simulink model "MicrogridControl"  (R2025b)
settings: Solver=VariableStepAuto  StartTime=0.0  StopTime=8  FixedStep=Ts  RelTol=1e-3
PreLoadFcn:
  | NormalOperation;
  | MicrogridControlParam;
undefined symbols (not defined in the file): base, bessModeInitial, bessSystem, bessVoltage, breakerStatus, DiscIntNeverNeededParam, ee_sli_rtmsupport, event, gcbh, generator, gflInverter, gfmInverter, Inertia, lineInductance, lineResistance, machine, plannedIsland, pmsm, powerLimit, powerQuality, PV, PVInverter, ref, resync, solar, solarInsolationChange, systemFrequency, Ts, windController, windSystem, windTurbine
libraries: nesl_utility x234, ee_lib x174, fl_lib x143, eeGeneralControl x137, simulink x78, eeTransforms x47, slpidlib x23, nesl_utility_internal x12, eePwmGenerator x9, eeSinusoidalMeasurementV2 x9, custom_lib x7, batteryecm_lib x6
(part 19 of 25)

== system MicrogridControl/Wind Farm/Wind Plant Integrated/Detailed/Wind Turbine and Converters/Wind Controller/Machine Converter Control/Power Controller ==
  windSpeed : Inport
  Derating Control : Subsystem
  Greater than : simulink/Logic and Bit Operations/Compare To Constant  relop=>  const=12  OutDataTypeStr=boolean
  Less than or equal to : simulink/Logic and Bit Operations/Compare To Constant  relop=<=  const=12  OutDataTypeStr=boolean
  Limiter Function Power Demand : Subsystem
  MPPT Control : Subsystem
  activePowerDemand : Outport
  wires:
  Limiter Function Power Demand/1(activePowerDemand) -> activePowerDemand/1
  Derating Control/1(activePowerDemand) -> Limiter Function Power Demand/2(activePowerDemandDerating)
  MPPT Control/1(activePowerDemand) -> Limiter Function Power Demand/1(activePowerDemandMPPT)
  Greater than/1 -> Derating Control/Enable
  Less than or equal to/1 -> MPPT Control/Enable
  windSpeed/1 -> MPPT Control/1(windSpeed), Less than or equal to/1, Greater than/1

== system MicrogridControl/Wind Farm/Wind Plant Integrated/Detailed/Wind Turbine and Converters/Wind Controller/Machine Converter Control/Subsystem ==
  note: LVRT Crowbar Control
  Vdc : Inport
  LVRT : Inport  Port=2
  Abs : Abs  SaturateOnIntegerOverflow=off
  Constant1 : Constant  Value=Vdc
  Product : Product
  Relay : Relay  OnSwitchValue=0.01001*Vdc  OffSwitchValue=0.01*Vdc
  Sum : Sum  Inputs=|+-
  Unit Delay1 : UnitDelay  SampleTime=-1  HasFrameUpgradeWarning=on
  Out1 : Outport
  wires:
  Relay/1 -> Out1/1
  Product/1 -> Abs/1
  LVRT/1 -> Product/2
  Unit Delay1/1 -> Sum/2
  Abs/1 -> Relay/1
  Sum/1 -> Product/1
  Vdc/1 -> Unit Delay1/1
  Constant1/1 -> Sum/1

== system MicrogridControl/Wind Farm/Wind Plant Integrated/Detailed/Wind Turbine and Converters/Wind Controller/Wind Grid-side Converter Controller/Current_controller ==
  iWindd : Inport
  iq : Inport  Port=2
  id-ref : Inport  Port=3
  iqref : Inport  Port=4
  Vd : Inport  Port=5
  Vq : Inport  Port=6
  Constant4 : Constant  Value=0
  Gain1 : Gain  Gain=2*1*pi*frequency*inductance/baseImpedance
  Gain2 : Gain  Gain=2*1*pi*frequency*inductance/baseImpedance
  Mux1 : Mux  Inputs=3
  PI : Subsystem
  PI1 : Subsystem
  Sum1 : Sum  Inputs=|+-
  Sum3 : Sum  Inputs=|++-
  Sum4 : Sum  Inputs=|+++
  Sum5 : Sum  Inputs=|+-
  Refrence_mdq0 : Outport
  wires:
  Mux1/1 -> Refrence_mdq0/1  "m_dqo"
  Sum4/1 -> [Eq], Mux1/2
  PI1/1(Out2) -> Sum4/1
  iqref/1 -> Sum5/1
  Sum5/1 -> PI1/1(Input)
  Constant4/1 -> Mux1/3
  Vd/1 -> Sum3/1
  Sum1/1 -> PI/1(Input)
  iq/1 -> Sum5/2, Gain2/1
  Vq/1 -> Sum4/2
  Gain1/1 -> Sum4/3
  id-ref/1 -> Sum1/1
  iWindd/1 -> Sum1/2, Gain1/1
  Gain2/1 -> Sum3/3
  Sum3/1 -> [Ed], Mux1/1
  PI/1(Out2) -> Sum3/2

== system MicrogridControl/Wind Farm/Wind Plant Integrated/Detailed/Wind Turbine and Converters/Wind Controller/Wind Grid-side Converter Controller/DC Bus Chopper control  ==
  note: LVRT Detection
  In1 : Inport
  Constant1 : Constant
  Constant2 : Constant  Value=0
  Switch : Switch  Criteria=u2 > Threshold  Threshold=0.9  SaturateOnIntegerOverflow=off  InputSameDT=off
  Unit Delay : UnitDelay  SampleTime=-1  HasFrameUpgradeWarning=on
  Out1 : Outport
  wires:
  Unit Delay/1 -> Switch/2
  In1/1 -> Unit Delay/1
  Constant2/1 -> Switch/1
  Constant1/1 -> Switch/3
  Switch/1 -> Out1/1

== system MicrogridControl/Wind Farm/Wind Plant Integrated/Detailed/Wind Turbine and Converters/Wind Controller/Wind Grid-side Converter Controller/DC voltage controller & current reference ==
  note: id_ref_generator
  note: iq_ref_generator
  note: Limiter
  Q_ref : Inport
  Vmag : Inport  Port=2
  Wind_Mpp_vdc : Inport  Port=3
  Wind_vdc : Inport  Port=4
  lvrt.iq : Inport  Port=5
  Constant : Constant
  Constant1 : Constant  Value=iMaxPU
  Current limits : Subsystem
  Scope : Scope  NumInputPorts=2
      settings: ActiveDisplayYMinimum=-1  ActiveDisplayYMaximum=1  DataLoggingVariableName=ScopeData32
  Scope1 : Scope
      settings: ActiveDisplayYMinimum=-1  ActiveDisplayYMaximum=1  DataLoggingVariableName=ScopeData37
  Scope2 : Scope  NumInputPorts=2
      settings: ActiveDisplayYMinimum=-1  ActiveDisplayYMaximum=1  DataLoggingVariableName=ScopeData38
  Subsystem : Subsystem
  Subsystem1 : Subsystem
  Switch : Switch  Criteria=u2 > Threshold  SaturateOnIntegerOverflow=off  InputSameDT=off
  Unit Delay1 : UnitDelay  SampleTime=Ts  HasFrameUpgradeWarning=on
  Unit Delay3 : UnitDelay  SampleTime=Ts  HasFrameUpgradeWarning=on
  id_ref : Outport
  iq_ref : Outport  Port=2
  wires:
  Constant/1 -> Switch/3
  Switch/1 -> Scope1/1, Subsystem/1(V_mag)
  Vmag/1 -> Switch/2, Switch/1
  lvrt.iq/1 -> Subsystem/3(lvrt.iq)
  Current limits/1(iubq) -> Scope2/1, Subsystem/2(iq_ub)
  Wind_vdc/1 -> Scope/2, Subsystem1/2(Wind_vdc)
  Q_ref/1 -> Subsystem/4(Q_ref)
  Unit Delay3/1 -> Current limits/3(idref)
  Subsystem1/1(Out1) -> Unit Delay3/1, id_ref/1
  Unit Delay1/1 -> Current limits/2(iqref)
  Constant1/1 -> Current limits/1(Imax)
  Subsystem/1(Out1) -> iq_ref/1, Unit Delay1/1
  Current limits/2(iubd) -> Scope2/2, Subsystem1/3(id_ub)
  Wind_Mpp_vdc/1 -> Scope/1, Subsystem1/1(Wind_Mpp_vdc)

== system MicrogridControl/Wind Farm/Wind Plant Integrated/Detailed/Wind Turbine and Converters/Wind Plant/Back-to-Back Converters/Average ==
  Chopper : Inport
  SM_ref : Inport  Port=2
  Grid_ref : Inport  Port=3
  Capacitor : fl_lib/Electrical/Electrical Elements/Capacitor  c=capDC F  r=1e-1 Ohm  g=0 1/Ohm  i_specify=off  i_priority=None  i=0 A  i_nominal_specify=off  i_nominal_value=1  i_nominal_unit=A  v_specify=off  v_priority=None  v=0 V  v_nominal_specify=off  v_nominal_value=1  v_nominal_unit=V  vc_specify=on  vc_priority=None  vc=Vdc V  vc_nominal_specify=off  vc_nominal_value=1  vc_nominal_unit=V
  Electrical Reference : fl_lib/Electrical/Electrical Elements/Electrical Reference
  Electrical Reference1 : fl_lib/Electrical/Electrical Elements/Electrical Reference
  Electrical Reference2 : fl_lib/Electrical/Electrical Elements/Electrical Reference
  Grid Side Converter : ee_lib/Semiconductors & Converters/Converters/Average-Value Voltage Source Converter (Three-Phase)  port_option=ee.enum.threePhasePort.composite  frequency_option=ee.enum.converters.frequency.variable  input_option=ee.enum.converters.inputOption.ModWave  FRated=60 Hz  losses_parameterization=ee.enum.converters.losses.fixed  Pfixed=1 W  ks=0.01  kc1=1.7 V  kc2=0.01 Ohm  Ploss_vect=[100, 800, 1870, 3250, 4900] W  Irms_vect=[10, 100, 200, 300, 400] A  Vdc_nom=300 V  thermal_mass=30000 J/K  temperature_specify=off  temperature_priority=High  temperature=298.15 K  temperature_nominal_specify=off  temperature_nominal_value=1  temperature_nominal_unit=K
      settings: InternalSimscapePortConfiguration="{\"Bottom\":[],\"Left\":[{\"id\":\"ModWave\",\"label\":\"ModWave\",\"type\":\"input\"},{\"id\":\"N\",\"label\":\"~\",\"type\":\"foundation.electrical.three_phase\"}],\"Right\":[{\"id\":\"p\",\"label\":\"+\",\"type\":\"foundation.electrical.electrical\"},{\"id\":\"n\",\"label\":\"-\",\"type\":\"foundation.electrical.electrical\"}],\"Top\":[]}"
  Ideal Semiconductor Switch : ee_lib/Semiconductors & Converters/Ideal Semiconductor Switch  port_option=ee.enum.controlport.ps  Ron=0.001 Ohm  Goff=1e-6 1/Ohm  Vth=0.5 V  diode_param=ee.enum.converters.protectiondiode.none  diode_Vf=0.8 V  diode_Ron=0.001 Ohm  diode_Goff=1e-5 1/Ohm  diode_C=50e-9 F  diode_iRM=-235 A  diode_iF=300 A  diode_idot=-50 A/us  diode_trr_param=ee.enum.converters.diodetrr.trr_factor  diode_trr_factor=3  diode_trr=15 us  diode_Qrr=1500 s*uA
  Machine Side Converter : ee_lib/Semiconductors & Converters/Converters/Average-Value Voltage Source Converter (Three-Phase)  port_option=ee.enum.threePhasePort.composite  frequency_option=ee.enum.converters.frequency.variable  input_option=ee.enum.converters.inputOption.ModWave  FRated=60 Hz  losses_parameterization=ee.enum.converters.losses.fixed  Pfixed=1 W  ks=0.01  kc1=1.7 V  kc2=0.01 Ohm  Ploss_vect=[100, 800, 1870, 3250, 4900] W  Irms_vect=[10, 100, 200, 300, 400] A  Vdc_nom=300 V  thermal_mass=30000 J/K  temperature_specify=off  temperature_priority=High  temperature=298.15 K  temperature_nominal_specify=off  temperature_nominal_value=1  temperature_nominal_unit=K
      settings: InternalSimscapePortConfiguration="{\"Bottom\":[],\"Left\":[{\"id\":\"ModWave\",\"label\":\"ModWave\",\"type\":\"input\"},{\"id\":\"N\",\"label\":\"~\",\"type\":\"foundation.electrical.three_phase\"}],\"Right\":[{\"id\":\"p\",\"label\":\"+\",\"type\":\"foundation.electrical.electrical\"},{\"id\":\"n\",\"label\":\"-\",\"type\":\"foundation.electrical.electrical\"}],\"Top\":[]}"
  PS-Simulink Converter1 : nesl_utility/PS-Simulink Converter  PhysicalDomain=network_engine_domain  SubClassName=ps_output  LeftPortType=input  RightPortType=output  PseudoPeriodic=off  Frequencies=[]  VectorFormat=1-D array  Unit=V  AffineConversion=off
  Resistor : fl_lib/Electrical/Electrical Elements/Resistor  R=16 Ohm  i_specify=off  i_priority=None  i=0 A  i_nominal_specify=off  i_nominal_value=1  i_nominal_unit=A  v_specify=off  v_priority=None  v=0 V  v_nominal_specify=off  v_nominal_value=1  v_nominal_unit=V
  Scope : Scope
      settings: ActiveDisplayYMinimum=-0.125  ActiveDisplayYMaximum=1.125  DataLoggingVariableName=ScopeData11
  Simulink-PS Converter : nesl_utility/Simulink-PS Converter  PhysicalDomain=network_engine_domain  SubClassName=ps_input  LeftPortType=input  RightPortType=output  PseudoPeriodic=off  Frequencies=[]  NoiseDistribution=none  NoiseParameters=[]  Unit=1  AffineConversion=off  FilteringAndDerivatives=provide  SimscapeFilterOrder=1  InputFilterTimeConstant=0.001  UdotUserProvided=0
  Simulink-PS Converter2 : nesl_utility/Simulink-PS Converter  PhysicalDomain=network_engine_domain  SubClassName=ps_input  LeftPortType=input  RightPortType=output  PseudoPeriodic=off  Frequencies=[]  NoiseDistribution=none  NoiseParameters=[]  Unit=1  AffineConversion=off  FilteringAndDerivatives=provide  SimscapeFilterOrder=1  InputFilterTimeConstant=0.001  UdotUserProvided=0
  Simulink-PS Converter4 : nesl_utility/Simulink-PS Converter  PhysicalDomain=network_engine_domain  SubClassName=ps_input  LeftPortType=input  RightPortType=output  PseudoPeriodic=off  Frequencies=[]  NoiseDistribution=none  NoiseParameters=[]  Unit=1  AffineConversion=off  FilteringAndDerivatives=provide  SimscapeFilterOrder=1  InputFilterTimeConstant=0.001  UdotUserProvided=0
  Voltage Sensor : fl_lib/Electrical/Electrical Sensors/Voltage Sensor
  In : PMIOPort  Side=Left
  ~ : PMIOPort  Port=2  Side=Right
  Vdc : Outport
  wires:
  SM_ref/1 -> Simulink-PS Converter/1
  PS-Simulink Converter1/1 -> Vdc/1  "Vdc"
  Chopper/1 -> Simulink-PS Converter2/1, Scope/1
  Grid_ref/1 -> Simulink-PS Converter4/1
  connections:
  Simulink-PS Converter/RConn1 -- Machine Side Converter/LConn1
  Machine Side Converter/LConn2 -- In/RConn1
  Simulink-PS Converter2/RConn1 -- Ideal Semiconductor Switch/LConn1
  Electrical Reference1/LConn1 -- Resistor/RConn1
  Grid Side Converter/LConn1 -- Simulink-PS Converter4/RConn1
  Resistor/LConn1 -- Ideal Semiconductor Switch/RConn2
  ~/RConn1 -- Grid Side Converter/LConn2
  PS-Simulink Converter1/LConn1 -- Voltage Sensor/RConn1
  Electrical Reference2/LConn1 -- Grid Side Converter/RConn2
  Voltage Sensor/LConn1 -- Machine Side Converter/RConn1 -- Ideal Semiconductor Switch/RConn1 -- Grid Side Converter/RConn1 -- Capacitor/LConn1
  Capacitor/RConn1 -- Voltage Sensor/RConn2 -- Machine Side Converter/RConn2 -- Electrical Reference/LConn1

== system MicrogridControl/Wind Farm/Wind Plant Integrated/Detailed/Wind Turbine and Converters/Wind Plant/Back-to-Back Converters/Switching ==
  Chopper : Inport
  SM_ref : Inport  Port=2
  Grid_ref : Inport  Port=3
  Capacitor : fl_lib/Electrical/Electrical Elements/Capacitor  c=capacitance F  r=1e-1 Ohm  g=0 1/Ohm  i_specify=off  i_priority=None  i=0 A  i_nominal_specify=off  i_nominal_value=1  i_nominal_unit=A  v_specify=off  v_priority=None  v=0 V  v_nominal_specify=off  v_nominal_value=1  v_nominal_unit=V  vc_specify=on  vc_priority=High  vc=baseVoltageDC V  vc_nominal_specify=off  vc_nominal_value=1  vc_nominal_unit=V
  Electrical Reference : fl_lib/Electrical/Electrical Elements/Electrical Reference
  Electrical Reference1 : fl_lib/Electrical/Electrical Elements/Electrical Reference
  Electrical Reference2 : fl_lib/Electrical/Electrical Elements/Electrical Reference
  Grid Side Converter : Subsystem
      settings: PortSchema="{\"entries\":[{\"content\":{\"sides\":[{\"content\":{\"connectorIds\":[\"LConn1\",\"LConn2\"]},\"type\":\"ConnectorPlacement.EquallySpacedRectSide\",\"uuid\":\"e32be008-cebd-46aa-ba62-c5c92b9b23e3\"},{\"content\":{\"connectorIds\":[\"In1\",\"RConn1\"],\"side\":\"RIGHT\"},\"type\":\"ConnectorPlacement.EquallySpacedRectSide\",\"uuid\":\"c483e451-04b5-4212-bdd1-c589ba5bea78\"},{\"content\":{\"side\":\"TOP\"},\"type\":\"ConnectorPlacement.EquallySpacedRectSide\",\"uuid\":\"824c135c-7e5f-4da0-a7de-e626b4bfa50d\"}]},\"type\":\"ConnectorPlacement.EquallySpacedConnector\",\"uuid\":\"5f81c72d-92ab-4525-91a6-193f769a7c86\"}],\"packageUris\":[\"http://schema.mathworks.com/mf0/Connector/R2020b\"],\"version\":\"1.0\"}"
  Ideal Semiconductor Switch : ee_lib/Semiconductors & Converters/Ideal Semiconductor Switch  port_option=ee.enum.controlport.ps  Ron=0.001 Ohm  Goff=1e-6 1/Ohm  Vth=0.5 V  diode_param=ee.enum.converters.protectiondiode.none  diode_Vf=0.8 V  diode_Ron=0.001 Ohm  diode_Goff=1e-5 1/Ohm  diode_C=50e-9 F  diode_iRM=-235 A  diode_iF=300 A  diode_idot=-50 A/us  diode_trr_param=ee.enum.converters.diodetrr.trr_factor  diode_trr_factor=3  diode_trr=15 us  diode_Qrr=1500 s*uA
  Machine Side Converter : Subsystem
      settings: PortSchema="{\"entries\":[{\"content\":{\"sides\":[{\"content\":{\"connectorIds\":[\"LConn1\",\"LConn2\"]},\"type\":\"ConnectorPlacement.EquallySpacedRectSide\",\"uuid\":\"e32be008-cebd-46aa-ba62-c5c92b9b23e3\"},{\"content\":{\"connectorIds\":[\"In1\",\"RConn1\"],\"side\":\"RIGHT\"},\"type\":\"ConnectorPlacement.EquallySpacedRectSide\",\"uuid\":\"c483e451-04b5-4212-bdd1-c589ba5bea78\"},{\"content\":{\"side\":\"TOP\"},\"type\":\"ConnectorPlacement.EquallySpacedRectSide\",\"uuid\":\"824c135c-7e5f-4da0-a7de-e626b4bfa50d\"}]},\"type\":\"ConnectorPlacement.EquallySpacedConnector\",\"uuid\":\"5f81c72d-92ab-4525-91a6-193f769a7c86\"}],\"packageUris\":[\"http://schema.mathworks.com/mf0/Connector/R2020b\"],\"version\":\"1.0\"}"
  PS-Simulink Converter1 : nesl_utility/PS-Simulink Converter  PhysicalDomain=network_engine_domain  SubClassName=ps_output  LeftPortType=input  RightPortType=output  PseudoPeriodic=off  Frequencies=[]  VectorFormat=1-D array  Unit=V  AffineConversion=off
  Resistor : fl_lib/Electrical/Electrical Elements/Resistor  R=16 Ohm  i_specify=off  i_priority=None  i=0 A  i_nominal_specify=off  i_nominal_value=1  i_nominal_unit=A  v_specify=off  v_priority=None  v=0 V  v_nominal_specify=off  v_nominal_value=1  v_nominal_unit=V
  Scope : Scope
      settings: ActiveDisplayYMinimum=-0.125  ActiveDisplayYMaximum=1.125  DataLoggingVariableName=ScopeData11
  Simulink-PS Converter2 : nesl_utility/Simulink-PS Converter  PhysicalDomain=network_engine_domain  SubClassName=ps_input  LeftPortType=input  RightPortType=output  PseudoPeriodic=off  Frequencies=[]  NoiseDistribution=none  NoiseParameters=[]  Unit=1  AffineConversion=off  FilteringAndDerivatives=provide  SimscapeFilterOrder=1  InputFilterTimeConstant=0.001  UdotUserProvided=0
  Voltage Sensor : fl_lib/Electrical/Electrical Sensors/Voltage Sensor
  In : PMIOPort  Side=Left
  ~ : PMIOPort  Port=2  Side=Right
  Vdc : Outport
  wires:
  PS-Simulink Converter1/1 -> Vdc/1  "Vdc"
  Chopper/1 -> Simulink-PS Converter2/1, Scope/1
  Grid_ref/1 -> Grid Side Converter/1(mabc)
  SM_ref/1 -> Machine Side Converter/1(mabc)
  connections:
  Machine Side Converter/RConn1 -- In/RConn1
  Simulink-PS Converter2/RConn1 -- Ideal Semiconductor Switch/LConn1
  Electrical Reference1/LConn1 -- Resistor/RConn1
  Resistor/LConn1 -- Ideal Semiconductor Switch/RConn2
  ~/RConn1 -- Grid Side Converter/RConn1
  PS-Simulink Converter1/LConn1 -- Voltage Sensor/RConn1
  Grid Side Converter/LConn2 -- Electrical Reference2/LConn1
  Voltage Sensor/LConn1 -- Machine Side Converter/LConn1 -- Capacitor/LConn1 -- Grid Side Converter/LConn1 -- Ideal Semiconductor Switch/RConn1
  Electrical Reference/LConn1 -- Voltage Sensor/RConn2 -- Machine Side Converter/LConn2 -- Capacitor/RConn1

== system MicrogridControl/Wind Farm/Wind Plant Integrated1/Detailed/Wind Turbine and Converters/Wind Controller/Machine Converter Control/Measurements ==
  iabc_sens : Inport
  w_sens : Inport  Port=2
  th_sens : Inport  Port=3
  Vdc_sens : Inport  Port=4
  2*pi : Constant  Value=2*pi  SampleTime=-1
  Math Function : Math  Operator=mod  SignedPower=on
  pole pairs : Gain  Gain=p
  "pole pairs " : Gain  Gain=p
  we : Outport  VectorParamsAs1DForOutWhenUnconnected=off
  iabc : Outport  Port=2  VectorParamsAs1DForOutWhenUnconnected=off
  theta : Outport  Port=3  VectorParamsAs1DForOutWhenUnconnected=off
  Vdc : Outport  Port=4  VectorParamsAs1DForOutWhenUnconnected=off
  wires:
  Math Function/1 -> theta/1
  Vdc_sens/1 -> Vdc/1
  "pole pairs "/1 -> Math Function/1
  th_sens/1 -> "pole pairs "/1
  2*pi/1 -> Math Function/2
  pole pairs/1 -> we/1
  iabc_sens/1 -> iabc/1
  w_sens/1 -> pole pairs/1

== system MicrogridControl/Wind Farm/Wind Plant Integrated1/Detailed/Wind Turbine and Converters/Wind Controller/Machine Converter Control/Power Controller ==
  windSpeed : Inport
  Derating Control : Subsystem
  Greater than : simulink/Logic and Bit Operations/Compare To Constant  relop=>  const=12  OutDataTypeStr=boolean
  Less than or equal to : simulink/Logic and Bit Operations/Compare To Constant  relop=<=  const=12  OutDataTypeStr=boolean
  Limiter Function Power Demand : Subsystem
  MPPT Control : Subsystem
  activePowerDemand : Outport
  wires:
  Limiter Function Power Demand/1(activePowerDemand) -> activePowerDemand/1
  Derating Control/1(activePowerDemand) -> Limiter Function Power Demand/2(activePowerDemandDerating)
  MPPT Control/1(activePowerDemand) -> Limiter Function Power Demand/1(activePowerDemandMPPT)
  Greater than/1 -> Derating Control/Enable
  Less than or equal to/1 -> MPPT Control/Enable
  windSpeed/1 -> MPPT Control/1(windSpeed), Less than or equal to/1, Greater than/1

== system MicrogridControl/Wind Farm/Wind Plant Integrated1/Detailed/Wind Turbine and Converters/Wind Controller/Machine Converter Control/Subsystem ==
  note: LVRT Crowbar Control
  Vdc : Inport
  LVRT : Inport  Port=2
  Abs : Abs  SaturateOnIntegerOverflow=off
  Constant1 : Constant  Value=Vdc
  Product : Product
  Relay : Relay  OnSwitchValue=0.01001*Vdc  OffSwitchValue=0.01*Vdc
  Sum : Sum  Inputs=|+-
  Unit Delay1 : UnitDelay  SampleTime=-1  HasFrameUpgradeWarning=on
  Out1 : Outport
  wires:
  Relay/1 -> Out1/1
  Product/1 -> Abs/1
  LVRT/1 -> Product/2
  Unit Delay1/1 -> Sum/2
  Abs/1 -> Relay/1
  Sum/1 -> Product/1
  Vdc/1 -> Unit Delay1/1
  Constant1/1 -> Sum/1

== system MicrogridControl/Wind Farm/Wind Plant Integrated1/Detailed/Wind Turbine and Converters/Wind Controller/Wind Grid-side Converter Controller/Current_controller ==
  iWindd : Inport
  iq : Inport  Port=2
  id-ref : Inport  Port=3
  iqref : Inport  Port=4
  Vd : Inport  Port=5
  Vq : Inport  Port=6
  Constant4 : Constant  Value=0
  Gain1 : Gain  Gain=2*1*pi*frequency*inductance/baseImpedance
  Gain2 : Gain  Gain=2*1*pi*frequency*inductance/baseImpedance
  Mux1 : Mux  Inputs=3
  PI : Subsystem
  PI1 : Subsystem
  Sum1 : Sum  Inputs=|+-
  Sum3 : Sum  Inputs=|++-
  Sum4 : Sum  Inputs=|+++
  Sum5 : Sum  Inputs=|+-
  Refrence_mdq0 : Outport
  wires:
  Mux1/1 -> Refrence_mdq0/1  "m_dqo"
  Sum4/1 -> [Eq], Mux1/2
  PI1/1(Out2) -> Sum4/1
  iqref/1 -> Sum5/1
  Sum5/1 -> PI1/1(Input)
  Constant4/1 -> Mux1/3
  Vd/1 -> Sum3/1
  Sum1/1 -> PI/1(Input)
  iq/1 -> Sum5/2, Gain2/1
  Vq/1 -> Sum4/2
  Gain1/1 -> Sum4/3
  id-ref/1 -> Sum1/1
  iWindd/1 -> Sum1/2, Gain1/1
  Gain2/1 -> Sum3/3
  Sum3/1 -> [Ed], Mux1/1
  PI/1(Out2) -> Sum3/2

== system MicrogridControl/Wind Farm/Wind Plant Integrated1/Detailed/Wind Turbine and Converters/Wind Controller/Wind Grid-side Converter Controller/DC Bus Chopper control  ==
  note: LVRT Detection
  In1 : Inport
  Constant1 : Constant
  Constant2 : Constant  Value=0
  Switch : Switch  Criteria=u2 > Threshold  Threshold=0.9  SaturateOnIntegerOverflow=off  InputSameDT=off
  Unit Delay : UnitDelay  SampleTime=-1  HasFrameUpgradeWarning=on
  Out1 : Outport
  wires:
  Unit Delay/1 -> Switch/2
  In1/1 -> Unit Delay/1
  Constant2/1 -> Switch/1
  Constant1/1 -> Switch/3
  Switch/1 -> Out1/1

== system MicrogridControl/Wind Farm/Wind Plant Integrated1/Detailed/Wind Turbine and Converters/Wind Controller/Wind Grid-side Converter Controller/DC voltage controller & current reference ==
  note: id_ref_generator
  note: iq_ref_generator
  note: Limiter
  Q_ref : Inport
  Vmag : Inport  Port=2
  Wind_Mpp_vdc : Inport  Port=3
  Wind_vdc : Inport  Port=4
  lvrt.iq : Inport  Port=5
  Constant : Constant
  Constant1 : Constant  Value=iMaxPU
  Current limits : Subsystem
  Subsystem : Subsystem
  Subsystem1 : Subsystem
  Switch : Switch  Criteria=u2 > Threshold  SaturateOnIntegerOverflow=off  InputSameDT=off
  Unit Delay1 : UnitDelay  SampleTime=Ts  HasFrameUpgradeWarning=on
  Unit Delay3 : UnitDelay  SampleTime=Ts  HasFrameUpgradeWarning=on
  id_ref : Outport
  iq_ref : Outport  Port=2
  wires:
  Constant/1 -> Switch/3
  Switch/1 -> Subsystem/1(V_mag)
  Vmag/1 -> Switch/2, Switch/1
  lvrt.iq/1 -> Subsystem/3(lvrt.iq)
  Current limits/1(iubq) -> Subsystem/2(iq_ub)
  Wind_vdc/1 -> Subsystem1/2(Wind_vdc)
  Wind_Mpp_vdc/1 -> Subsystem1/1(Wind_Mpp_vdc)
  Q_ref/1 -> Subsystem/4(Q_ref)
  Unit Delay3/1 -> Current limits/3(idref)
  Subsystem1/1(Out1) -> Unit Delay3/1, id_ref/1
  Unit Delay1/1 -> Current limits/2(iqref)
  Constant1/1 -> Current limits/1(Imax)
  Subsystem/1(Out1) -> iq_ref/1, Unit Delay1/1
  Current limits/2(iubd) -> Subsystem1/3(id_ub)

== system MicrogridControl/Wind Farm/Wind Plant Integrated1/Detailed/Wind Turbine and Converters/Wind Plant/Back-to-Back Converters/Average ==
  Chopper : Inport
  SM_ref : Inport  Port=2
  Grid_ref : Inport  Port=3
  Capacitor : fl_lib/Electrical/Electrical Elements/Capacitor  c=capDC F  r=1e-1 Ohm  g=0 1/Ohm  i_specify=off  i_priority=None  i=0 A  i_nominal_specify=off  i_nominal_value=1  i_nominal_unit=A  v_specify=off  v_priority=None  v=0 V  v_nominal_specify=off  v_nominal_value=1  v_nominal_unit=V  vc_specify=on  vc_priority=None  vc=Vdc V  vc_nominal_specify=off  vc_nominal_value=1  vc_nominal_unit=V
  Electrical Reference : fl_lib/Electrical/Electrical Elements/Electrical Reference
  Electrical Reference1 : fl_lib/Electrical/Electrical Elements/Electrical Reference
  Electrical Reference2 : fl_lib/Electrical/Electrical Elements/Electrical Reference
  Grid Side Converter : ee_lib/Semiconductors & Converters/Converters/Average-Value Voltage Source Converter (Three-Phase)  port_option=ee.enum.threePhasePort.composite  frequency_option=ee.enum.converters.frequency.variable  input_option=ee.enum.converters.inputOption.ModWave  FRated=60 Hz  losses_parameterization=ee.enum.converters.losses.fixed  Pfixed=1 W  ks=0.01  kc1=1.7 V  kc2=0.01 Ohm  Ploss_vect=[100, 800, 1870, 3250, 4900] W  Irms_vect=[10, 100, 200, 300, 400] A  Vdc_nom=300 V  thermal_mass=30000 J/K  temperature_specify=off  temperature_priority=High  temperature=298.15 K  temperature_nominal_specify=off  temperature_nominal_value=1  temperature_nominal_unit=K
      settings: InternalSimscapePortConfiguration="{\"Bottom\":[],\"Left\":[{\"id\":\"ModWave\",\"label\":\"ModWave\",\"type\":\"input\"},{\"id\":\"N\",\"label\":\"~\",\"type\":\"foundation.electrical.three_phase\"}],\"Right\":[{\"id\":\"p\",\"label\":\"+\",\"type\":\"foundation.electrical.electrical\"},{\"id\":\"n\",\"label\":\"-\",\"type\":\"foundation.electrical.electrical\"}],\"Top\":[]}"
  Ideal Semiconductor Switch : ee_lib/Semiconductors & Converters/Ideal Semiconductor Switch  port_option=ee.enum.controlport.ps  Ron=0.001 Ohm  Goff=1e-6 1/Ohm  Vth=0.5 V  diode_param=ee.enum.converters.protectiondiode.none  diode_Vf=0.8 V  diode_Ron=0.001 Ohm  diode_Goff=1e-5 1/Ohm  diode_C=50e-9 F  diode_iRM=-235 A  diode_iF=300 A  diode_idot=-50 A/us  diode_trr_param=ee.enum.converters.diodetrr.trr_factor  diode_trr_factor=3  diode_trr=15 us  diode_Qrr=1500 s*uA
  Machine Side Converter : ee_lib/Semiconductors & Converters/Converters/Average-Value Voltage Source Converter (Three-Phase)  port_option=ee.enum.threePhasePort.composite  frequency_option=ee.enum.converters.frequency.variable  input_option=ee.enum.converters.inputOption.ModWave  FRated=60 Hz  losses_parameterization=ee.enum.converters.losses.fixed  Pfixed=1 W  ks=0.01  kc1=1.7 V  kc2=0.01 Ohm  Ploss_vect=[100, 800, 1870, 3250, 4900] W  Irms_vect=[10, 100, 200, 300, 400] A  Vdc_nom=300 V  thermal_mass=30000 J/K  temperature_specify=off  temperature_priority=High  temperature=298.15 K  temperature_nominal_specify=off  temperature_nominal_value=1  temperature_nominal_unit=K
      settings: InternalSimscapePortConfiguration="{\"Bottom\":[],\"Left\":[{\"id\":\"ModWave\",\"label\":\"ModWave\",\"type\":\"input\"},{\"id\":\"N\",\"label\":\"~\",\"type\":\"foundation.electrical.three_phase\"}],\"Right\":[{\"id\":\"p\",\"label\":\"+\",\"type\":\"foundation.electrical.electrical\"},{\"id\":\"n\",\"label\":\"-\",\"type\":\"foundation.electrical.electrical\"}],\"Top\":[]}"
  PS-Simulink Converter1 : nesl_utility/PS-Simulink Converter  PhysicalDomain=network_engine_domain  SubClassName=ps_output  LeftPortType=input  RightPortType=output  PseudoPeriodic=off  Frequencies=[]  VectorFormat=1-D array  Unit=V  AffineConversion=off
  Resistor : fl_lib/Electrical/Electrical Elements/Resistor  R=16 Ohm  i_specify=off  i_priority=None  i=0 A  i_nominal_specify=off  i_nominal_value=1  i_nominal_unit=A  v_specify=off  v_priority=None  v=0 V  v_nominal_specify=off  v_nominal_value=1  v_nominal_unit=V
  Scope : Scope
      settings: ActiveDisplayYMinimum=-0.125  ActiveDisplayYMaximum=1.125  DataLoggingVariableName=ScopeData11
  Simulink-PS Converter : nesl_utility/Simulink-PS Converter  PhysicalDomain=network_engine_domain  SubClassName=ps_input  LeftPortType=input  RightPortType=output  PseudoPeriodic=off  Frequencies=[]  NoiseDistribution=none  NoiseParameters=[]  Unit=1  AffineConversion=off  FilteringAndDerivatives=provide  SimscapeFilterOrder=1  InputFilterTimeConstant=0.001  UdotUserProvided=0
  Simulink-PS Converter2 : nesl_utility/Simulink-PS Converter  PhysicalDomain=network_engine_domain  SubClassName=ps_input  LeftPortType=input  RightPortType=output  PseudoPeriodic=off  Frequencies=[]  NoiseDistribution=none  NoiseParameters=[]  Unit=1  AffineConversion=off  FilteringAndDerivatives=provide  SimscapeFilterOrder=1  InputFilterTimeConstant=0.001  UdotUserProvided=0
  Simulink-PS Converter4 : nesl_utility/Simulink-PS Converter  PhysicalDomain=network_engine_domain  SubClassName=ps_input  LeftPortType=input  RightPortType=output  PseudoPeriodic=off  Frequencies=[]  NoiseDistribution=none  NoiseParameters=[]  Unit=1  AffineConversion=off  FilteringAndDerivatives=provide  SimscapeFilterOrder=1  InputFilterTimeConstant=0.001  UdotUserProvided=0
  Voltage Sensor : fl_lib/Electrical/Electrical Sensors/Voltage Sensor
  In : PMIOPort  Side=Left
  ~ : PMIOPort  Port=2  Side=Right
  Vdc : Outport
  wires:
  SM_ref/1 -> Simulink-PS Converter/1
  PS-Simulink Converter1/1 -> Vdc/1  "Vdc"
  Chopper/1 -> Simulink-PS Converter2/1, Scope/1
  Grid_ref/1 -> Simulink-PS Converter4/1
  connections:
  Simulink-PS Converter/RConn1 -- Machine Side Converter/LConn1
  Machine Side Converter/LConn2 -- In/RConn1
  Simulink-PS Converter2/RConn1 -- Ideal Semiconductor Switch/LConn1
  Electrical Reference1/LConn1 -- Resistor/RConn1
  Grid Side Converter/LConn1 -- Simulink-PS Converter4/RConn1
  Resistor/LConn1 -- Ideal Semiconductor Switch/RConn2
  ~/RConn1 -- Grid Side Converter/LConn2
  PS-Simulink Converter1/LConn1 -- Voltage Sensor/RConn1
  Electrical Reference2/LConn1 -- Grid Side Converter/RConn2
  Voltage Sensor/LConn1 -- Machine Side Converter/RConn1 -- Ideal Semiconductor Switch/RConn1 -- Grid Side Converter/RConn1 -- Capacitor/LConn1
  Capacitor/RConn1 -- Voltage Sensor/RConn2 -- Machine Side Converter/RConn2 -- Electrical Reference/LConn1

== system MicrogridControl/Wind Farm/Wind Plant Integrated1/Detailed/Wind Turbine and Converters/Wind Plant/Back-to-Back Converters/Switching ==
  Chopper : Inport
  SM_ref : Inport  Port=2
  Grid_ref : Inport  Port=3
  Capacitor : fl_lib/Electrical/Electrical Elements/Capacitor  c=capacitance F  r=1e-1 Ohm  g=0 1/Ohm  i_specify=off  i_priority=None  i=0 A  i_nominal_specify=off  i_nominal_value=1  i_nominal_unit=A  v_specify=off  v_priority=None  v=0 V  v_nominal_specify=off  v_nominal_value=1  v_nominal_unit=V  vc_specify=on  vc_priority=High  vc=baseVoltageDC V  vc_nominal_specify=off  vc_nominal_value=1  vc_nominal_unit=V
  Electrical Reference : fl_lib/Electrical/Electrical Elements/Electrical Reference
  Electrical Reference1 : fl_lib/Electrical/Electrical Elements/Electrical Reference
  Electrical Reference2 : fl_lib/Electrical/Electrical Elements/Electrical Reference
  Grid Side Converter : Subsystem
      settings: PortSchema="{\"entries\":[{\"content\":{\"sides\":[{\"content\":{\"connectorIds\":[\"LConn1\",\"LConn2\"]},\"type\":\"ConnectorPlacement.EquallySpacedRectSide\",\"uuid\":\"e32be008-cebd-46aa-ba62-c5c92b9b23e3\"},{\"content\":{\"connectorIds\":[\"In1\",\"RConn1\"],\"side\":\"RIGHT\"},\"type\":\"ConnectorPlacement.EquallySpacedRectSide\",\"uuid\":\"c483e451-04b5-4212-bdd1-c589ba5bea78\"},{\"content\":{\"side\":\"TOP\"},\"type\":\"ConnectorPlacement.EquallySpacedRectSide\",\"uuid\":\"824c135c-7e5f-4da0-a7de-e626b4bfa50d\"}]},\"type\":\"ConnectorPlacement.EquallySpacedConnector\",\"uuid\":\"5f81c72d-92ab-4525-91a6-193f769a7c86\"}],\"packageUris\":[\"http://schema.mathworks.com/mf0/Connector/R2020b\"],\"version\":\"1.0\"}"
  Ideal Semiconductor Switch : ee_lib/Semiconductors & Converters/Ideal Semiconductor Switch  port_option=ee.enum.controlport.ps  Ron=0.001 Ohm  Goff=1e-6 1/Ohm  Vth=0.5 V  diode_param=ee.enum.converters.protectiondiode.none  diode_Vf=0.8 V  diode_Ron=0.001 Ohm  diode_Goff=1e-5 1/Ohm  diode_C=50e-9 F  diode_iRM=-235 A  diode_iF=300 A  diode_idot=-50 A/us  diode_trr_param=ee.enum.converters.diodetrr.trr_factor  diode_trr_factor=3  diode_trr=15 us  diode_Qrr=1500 s*uA
  Machine Side Converter : Subsystem
      settings: PortSchema="{\"entries\":[{\"content\":{\"sides\":[{\"content\":{\"connectorIds\":[\"LConn1\",\"LConn2\"]},\"type\":\"ConnectorPlacement.EquallySpacedRectSide\",\"uuid\":\"e32be008-cebd-46aa-ba62-c5c92b9b23e3\"},{\"content\":{\"connectorIds\":[\"In1\",\"RConn1\"],\"side\":\"RIGHT\"},\"type\":\"ConnectorPlacement.EquallySpacedRectSide\",\"uuid\":\"c483e451-04b5-4212-bdd1-c589ba5bea78\"},{\"content\":{\"side\":\"TOP\"},\"type\":\"ConnectorPlacement.EquallySpacedRectSide\",\"uuid\":\"824c135c-7e5f-4da0-a7de-e626b4bfa50d\"}]},\"type\":\"ConnectorPlacement.EquallySpacedConnector\",\"uuid\":\"5f81c72d-92ab-4525-91a6-193f769a7c86\"}],\"packageUris\":[\"http://schema.mathworks.com/mf0/Connector/R2020b\"],\"version\":\"1.0\"}"
  PS-Simulink Converter1 : nesl_utility/PS-Simulink Converter  PhysicalDomain=network_engine_domain  SubClassName=ps_output  LeftPortType=input  RightPortType=output  PseudoPeriodic=off  Frequencies=[]  VectorFormat=1-D array  Unit=V  AffineConversion=off
  Resistor : fl_lib/Electrical/Electrical Elements/Resistor  R=16 Ohm  i_specify=off  i_priority=None  i=0 A  i_nominal_specify=off  i_nominal_value=1  i_nominal_unit=A  v_specify=off  v_priority=None  v=0 V  v_nominal_specify=off  v_nominal_value=1  v_nominal_unit=V
  Scope : Scope
      settings: ActiveDisplayYMinimum=-0.125  ActiveDisplayYMaximum=1.125  DataLoggingVariableName=ScopeData11
  Simulink-PS Converter2 : nesl_utility/Simulink-PS Converter  PhysicalDomain=network_engine_domain  SubClassName=ps_input  LeftPortType=input  RightPortType=output  PseudoPeriodic=off  Frequencies=[]  NoiseDistribution=none  NoiseParameters=[]  Unit=1  AffineConversion=off  FilteringAndDerivatives=provide  SimscapeFilterOrder=1  InputFilterTimeConstant=0.001  UdotUserProvided=0
  Voltage Sensor : fl_lib/Electrical/Electrical Sensors/Voltage Sensor
  In : PMIOPort  Side=Left
  ~ : PMIOPort  Port=2  Side=Right
  Vdc : Outport
  wires:
  PS-Simulink Converter1/1 -> Vdc/1  "Vdc"
  Chopper/1 -> Simulink-PS Converter2/1, Scope/1
  Grid_ref/1 -> Grid Side Converter/1(mabc)
  SM_ref/1 -> Machine Side Converter/1(mabc)
  connections:
  Machine Side Converter/RConn1 -- In/RConn1
  Simulink-PS Converter2/RConn1 -- Ideal Semiconductor Switch/LConn1
  Electrical Reference1/LConn1 -- Resistor/RConn1
  Resistor/LConn1 -- Ideal Semiconductor Switch/RConn2
  ~/RConn1 -- Grid Side Converter/RConn1
  PS-Simulink Converter1/LConn1 -- Voltage Sensor/RConn1
  Grid Side Converter/LConn2 -- Electrical Reference2/LConn1
  Voltage Sensor/LConn1 -- Machine Side Converter/LConn1 -- Capacitor/LConn1 -- Grid Side Converter/LConn1 -- Ideal Semiconductor Switch/RConn1
  Electrical Reference/LConn1 -- Voltage Sensor/RConn2 -- Machine Side Converter/LConn2 -- Capacitor/RConn1

== system MicrogridControl/BESS/BESS Integrated/Detailed/BESS Controller/Grid Forming/Current Limiting/CurrentLimitingMethod/currentLimitAndVirtual ==
  Igd : Inport
  Igq : Inport  Port=2
  Current Saturation : Subsystem
  CurrentLimitSelection : Stateflow chart  TreatAsAtomicUnit=on
  Math Function : Math  Operator=hypot
  Merge{,1..3} (4 alike) : Merge  Inputs=3
  No Fault Ride Through : Subsystem
  VI : Subsystem
  delVd : Outport
  delVq : Outport  Port=2
  Idmax : Outport  Port=3
  Iqmax : Outport  Port=4
  wires:
  [Imax] -> VI/3(Imax)
  [Imax] -> Current Saturation/3(Imaxsat)
  [noCtLt] -> No Fault Ride Through/Enable
  [satCtLt] -> Current Saturation/Enable
  [viCtLt] -> VI/Enable
  CurrentLimitSelection/4(satCurrentLimit) -> [satCtLt]
  CurrentLimitSelection/3(viCurrentLimit) -> [viCtLt]
  CurrentLimitSelection/2(noCurrentLimit) -> [noCtLt]
  CurrentLimitSelection/1(ismax) -> [Imax]
  Math Function/1 -> CurrentLimitSelection/1(Is)
  No Fault Ride Through/2(delVq) -> Merge1/3
  Merge3/1 -> Iqmax/1
  Current Saturation/2(delVq) -> Merge1/2
  No Fault Ride Through/4(iqmax) -> Merge3/3
  VI/3(idmax) -> Merge2/1
  VI/4(iqmax) -> Merge3/1
  Current Saturation/3(idmax) -> Merge2/2
  VI/2(delVq) -> Merge1/1
  Merge/1 -> delVd/1
  Current Saturation/4(iqmax) -> Merge3/2
  Current Saturation/1(delVd) -> Merge/2
  [Id] -> Math Function/1
  [Iq] -> Math Function/2
  VI/1(delVd) -> Merge/1
  No Fault Ride Through/3(idmax) -> Merge2/3
  No Fault Ride Through/1(delVd) -> Merge/3
  Igd/1 -> [Id], No Fault Ride Through/1(Id), Current Saturation/1(Id), VI/1(Id)
  Merge1/1 -> delVq/1
  Igq/1 -> [Iq], No Fault Ride Through/2(Iq), VI/2(Iq), Current Saturation/2(Iq)
  Merge2/1 -> Idmax/1

== system MicrogridControl/BESS/BESS Integrated/Detailed/BESS Controller/Grid Forming/Current Limiting/CurrentLimitingMethod/currentSaturation ==
  note: Vs-delV
  Igd : Inport
  Igq : Inport  Port=2
  Compare : Subsystem
  Constant : Constant  Value=maxSatCurrentLimit
  Constant1 : Constant  Value=0
  Constant2 : Constant  Value=0
  If : If
  If Action Subsystem : Subsystem  TreatAsAtomicUnit=on
  If Action Subsystem1 : Subsystem  TreatAsAtomicUnit=on
  Math Function : Math  Operator=hypot
  Merge : Merge
  Merge1 : Merge
  Subtract : Sum  Inputs=+-
  delVd : Outport
  delVq : Outport  Port=2
  Idmax : Outport  Port=3
  Iqmax : Outport  Port=4
  wires:
  Merge1/1 -> Iqmax/1
  Merge/1 -> Idmax/1
  Constant1/1 -> delVd/1
  Constant2/1 -> delVq/1
  If Action Subsystem1/2(Iqmax) -> Merge1/2
  If Action Subsystem/2(Iqmax) -> Merge1/1
  If Action Subsystem1/1(Idmax) -> Merge/2
  If Action Subsystem/1(Idmax) -> Merge/1
  [Is] -> If Action Subsystem/1(Is)
  If/2 -> If Action Subsystem1/Action
  Compare/1(Out1) -> If/1
  Subtract/1 -> Compare/1(u)
  [Isq] -> If Action Subsystem/3(Isq)
  [Isd] -> If Action Subsystem/2(Isd)
  If/1 -> If Action Subsystem/Action
  Math Function/1 -> Subtract/2, [Is]  "Is"
  Constant/1 -> Subtract/1
  Igq/1 -> Math Function/2, [Isq]
  Igd/1 -> Math Function/1, [Isd]

== system MicrogridControl/BESS/BESS Integrated/Detailed/BESS Controller/Grid Forming/Current Limiting/CurrentLimitingMethod/virtualImpedance ==
  note: Resistance coefficient
  note: X/R ratio
  Igd : Inport
  Igq : Inport  Port=2
  Constant : Constant  Value=maxVICurrentLimit
  Constant1 : Constant  Value=0
  Constant2 : Constant  Value=0
  Constant3 : Constant  Value=0
  Gain : Gain  Gain=ctLimitVirtualImp
  Gain1 : Gain  Gain=ctLimitXbyR
  Low-Pass Filter : eeGeneralControl/Low-Pass Filter (Discrete or Continuous)  K=1  T=currentVITimeConst  B=inf  A=-inf  init_option=Inherited from block input  x0=0  Ts=-1
  Math Function : Math  Operator=hypot
  Product{,1..3} (4 alike) : Product
  Relay : Relay  OnSwitchValue=0.01  OffSwitchValue=-0.05
  Saturation : Saturate  UpperLimit=1  LowerLimit=-1
  Saturation1 : Saturate  UpperLimit=1  LowerLimit=-1
  Sum : Sum  Inputs=|+-
  Sum1 : Sum  Inputs=|+-
  Sum2 : Sum  Inputs=++|
  Switch : Switch  Criteria=u2 > Threshold  SaturateOnIntegerOverflow=off  InputSameDT=off
  delVd : Outport
  delVq : Outport  Port=2
  Idmax : Outport  Port=3
  Iqmax : Outport  Port=4
  wires:
  Sum2/1 -> Saturation1/1
  Product3/1 -> Sum2/2
  Low-Pass Filter/1 -> Sum/1
  Saturation/1 -> delVd/1
  Relay/1 -> Switch/2
  Saturation1/1 -> delVq/1
  Igd/1 -> [Igd], Math Function/1
  Constant1/1 -> Switch/3
  Gain/1 -> Switch/1
  Constant3/1 -> Iqmax/1
  Constant2/1 -> Idmax/1
  [Igd] -> Product/2, Product1/1
  Switch/1 -> Product/1, Product3/2, Gain1/1
  [Igq] -> Product2/2, Product3/1
  Math Function/1 -> Low-Pass Filter/1  "Is"
  Constant/1 -> Sum/2  "IsMaxium"
  Product2/1 -> Sum1/2
  Product/1 -> Sum1/1
  Sum1/1 -> Saturation/1
  Gain1/1 -> Product2/1, Product1/2
  Product1/1 -> Sum2/1
  Igq/1 -> Math Function/2, [Igq]
  Sum/1 -> Relay/1, Gain/1

== system MicrogridControl/BESS/BESS Integrated/Detailed/BESS Controller/Grid Forming/Grid Voltage Reactive Power Support/Modifying Active Power Reference/Computing New Active Power Ref ==
  Iq : Inport
  Vd : Inport  Port=2
  Abs : Abs  SaturateOnIntegerOverflow=off
  Constant : Constant  Value=maxVICurrentLimit*0.96
  Constant1 : Constant  Value=0
  Product : Product
  Sqrt : Sqrt
  Square : Math  Operator=square
  Square1 : Math  Operator=square
  Subtract : Sum  Inputs=-+
  Switch : Switch  Criteria=u2 > Threshold  Threshold=1.15  SaturateOnIntegerOverflow=off  InputSameDT=off
  Pref : Outport
  wires:
  Product/1 -> Pref/1
  Iq/1 -> Square/1
  Sqrt/1 -> Abs/1
  Vd/1 -> Product/1
  Constant1/1 -> Switch/1
  Square1/1 -> Subtract/2
  Square/1 -> Switch/2, Subtract/1
  Switch/1 -> Product/2
  Subtract/1 -> Sqrt/1
  Constant/1 -> Square1/1
  Abs/1 -> Switch/3

== system MicrogridControl/BESS/BESS Integrated/Detailed/BESS Controller/Grid Forming/Grid Voltage Reactive Power Support/Modifying Reactive Power Reference/Changing the Power Reference ==
  Vs : Inport
  Vd : Inport  Port=2
  Pref : Inport  Port=3
  Qref : Inport  Port=4
  Enable : EnablePort
  ActivePowerReference : Subsystem
  Constant1 : Constant  Value=voltreference*0.96
  EstimateIdForGivenIq : Subsystem
  EstimateIqForReactivePower : Subsystem
  Max : MinMax  Function=max  Inputs=2
  ReactivePowerReference : Subsystem
  Prefv : Outport
  Qrefv : Outport  Port=2
  wires:
  Vd/1 -> EstimateIqForReactivePower/2(Vd)
  Qref/1 -> Max/2
  ReactivePowerReference/1(QrefNew) -> Max/1
  Pref/1 -> ActivePowerReference/3(Pref)
  EstimateIdForGivenIq/1(Id) -> ActivePowerReference/1(Id)
  Vs/1 -> ReactivePowerReference/1(Vd), EstimateIqForReactivePower/3(Vs), ActivePowerReference/2(Vd)
  Constant1/1 -> EstimateIqForReactivePower/1(Vmin)
  EstimateIqForReactivePower/1(Iq) -> ReactivePowerReference/2(Iq), EstimateIdForGivenIq/1(Iq)
  Max/1 -> Qrefv/1
  ActivePowerReference/1(PrefNew) -> Prefv/1

== system MicrogridControl/BESS/BESS Integrated/Detailed/BESS Controller/Grid Forming/Grid Voltage Reactive Power Support/Modifying Reactive Power Reference/Hysteresis ==
  Vs : Inport
  AND : Logic  IconShape=distinctive  AllPortsSameDT=off  OutDataTypeStr=boolean
  Compare To Constant : simulink/Logic and Bit Operations/Compare To Constant  relop=<  const=0.9  OutDataTypeStr=boolean
  Compare To Constant1 : simulink/Logic and Bit Operations/Compare To Constant  relop=<  const=0.95  OutDataTypeStr=boolean
  D Latch : simulink_extras/Flip Flops/D Latch
  OR : Logic  Operator=OR  IconShape=distinctive  AllPortsSameDT=off  OutDataTypeStr=boolean
  Scope : Scope
      settings: ActiveDisplayYMinimum=0.96929  ActiveDisplayYMaximum=1.01111
  Terminator : Terminator
  LVFlag : Outport
  wires:
  Vs/1 -> Compare To Constant/1, Compare To Constant1/1, Scope/1
  Compare To Constant/1 -> OR/2, D Latch/2, D Latch/1
  D Latch/2 -> Terminator/1
  OR/1 -> LVFlag/1
  AND/1 -> OR/1
  D Latch/1 -> AND/2
  Compare To Constant1/1 -> AND/1

== system MicrogridControl/BESS/BESS Integrated/Detailed/BESS Controller/Grid Forming/Grid Voltage Reactive Power Support/Modifying Reactive Power Reference/Not Altering the Power Reference ==
  Pref : Inport
  Qref : Inport  Port=2
  Enable : EnablePort
  Prefv : Outport
  Qrefv : Outport  Port=2
  wires:
  Qref/1 -> Qrefv/1
  Pref/1 -> Prefv/1

== system MicrogridControl/BESS/BESS Integrated/Detailed/BESS Controller/Grid Forming/Measurement/Frequency Measurement/Frequency Measurement ==
  abc : Inport
  Constant : Constant
  Discrete-Time Integrator : DiscreteIntegrator  SampleTime=sampleTime  LimitOutput=on  ICPrevOutput=DiscIntNeverNeededParam  ICPrevScaledInput=DiscIntNeverNeededParam
  If : If  IfExpression=u1 > 0.9
  If Action Subsystem : Subsystem  TreatAsAtomicUnit=on
  If Action Subsystem1 : Subsystem  TreatAsAtomicUnit=on
  Merge : Merge
  Postive Sequence : Subsystem
  Freq : Outport
  wires:
  Postive Sequence/1(posSeq) -> If Action Subsystem/1(V)
  Merge/1 -> Freq/1
  If Action Subsystem1/1(Out1) -> Merge/2
  If Action Subsystem/1(Freq) -> Merge/1
  Constant/1 -> Discrete-Time Integrator/1
  abc/1 -> Postive Sequence/1(abc)
  Discrete-Time Integrator/1 -> If/1, If Action Subsystem/2(Time)
  If/2 -> If Action Subsystem1/Action
  If/1 -> If Action Subsystem/Action

== system MicrogridControl/BESS/BESS Integrated/Detailed/BESS Controller/Grid Forming/Measurement/abc2dq/Supply Current to dq ==
  abc : Inport
  Angle : Inport  Port=2
  Demux : Demux  Outputs=3
  Park Transform : eeTransforms/Park Transform  AxisAlignment=D-axis  PowerInvariant=off
  Terminator : Terminator
  Igd : Outport  VectorParamsAs1DForOutWhenUnconnected=off
  Igq : Outport  Port=2  VectorParamsAs1DForOutWhenUnconnected=off
  wires:
  Angle/1 -> Park Transform/2
  abc/1 -> Park Transform/1
  Demux/1 -> Igd/1
  Demux/2 -> Igq/1
  Park Transform/1 -> Demux/1
  Demux/3 -> Terminator/1

== system MicrogridControl/BESS/BESS Integrated/Detailed/BESS Controller/Grid Forming/Measurement/abc2dq/Supply Voltage  to dq1 ==
  Angle : Inport
  abc : Inport  Port=2
  Demux : Demux  Outputs=3
  Park Transform : eeTransforms/Park Transform  AxisAlignment=D-axis  PowerInvariant=off
  Terminator : Terminator
  Vgd : Outport  VectorParamsAs1DForOutWhenUnconnected=off
  Vgq : Outport  Port=2  VectorParamsAs1DForOutWhenUnconnected=off
  wires:
  Angle/1 -> Park Transform/2
  abc/1 -> Park Transform/1
  Demux/1 -> Vgd/1
  Demux/2 -> Vgq/1
  Park Transform/1 -> Demux/1
  Demux/3 -> Terminator/1

== system MicrogridControl/BESS/BESS Integrated/Detailed/BESS Controller/Grid Forming/Power Control/ActivePowerControl/droopControl ==
  Pref : Inport
  Pmeas : Inport  Port=2
  fref : Inport  Port=3
  cntrlflag : Inport  Port=4
  fgrid : Inport  Port=5
  Add : Sum  Inputs=+-
  Constant : Constant
  Constant5 : Constant  Value=pi/2
  Gain : Gain  Gain=powerFreq*2*pi
  Integrator with Wrapped State (Discrete or Continuous) : eeGeneralControl/Integrator with Wrapped State (Discrete or Continuous)  LabelModeActiveChoice=Discrete  WrappedStateUpperValue=2*pi  WrappedStateLowerValue=0  x0=0  Ts=activePowerSampleTime
  Lead-Lag (Discrete or Continuous) : eeGeneralControl/Lead-Lag (Discrete or Continuous)  T1=droopT1  T2=droopT2  B=inf  A=-inf  init_option=Inherited from block input  x0=0  Ts=activePowerSampleTime
  Low-Pass Filter (Discrete or Continuous) : eeGeneralControl/Low-Pass Filter (Discrete or Continuous)  K=1  T=droopTC  B=inf  A=-inf  init_option=Specify as parameter  x0=0  Ts=activePowerSampleTime
  Scope : Scope
  Scope1 : Scope
  Scope2 : Scope
  Sum : Sum  Inputs=|-+
  Sum1 : Sum  Inputs=|-+
  Terminator : Terminator
  Terminator1 : Terminator
  Terminator2 : Terminator
  mp : Gain  Gain=droopSlope
  Theta : Outport
  w : Outport  Port=2
  wires:
  cntrlflag/1 -> Terminator2/1
  fref/1 -> Terminator1/1
  fgrid/1 -> Terminator/1
  Sum1/1 -> Gain/1
  Constant/1 -> Sum1/2
  Integrator with Wrapped State (Discrete or Continuous)/1 -> Add/1
  Lead-Lag (Discrete or Continuous)/1 -> Sum/2
  Gain/1 -> w/1, Integrator with Wrapped State (Discrete or Continuous)/1
  Pref/1 -> Sum/1
  Constant5/1 -> Add/2
  Add/1 -> Theta/1, Scope1/1
  Pmeas/1 -> Lead-Lag (Discrete or Continuous)/1
  Sum/1 -> mp/1, Scope/1
  mp/1 -> Low-Pass Filter (Discrete or Continuous)/1
  Low-Pass Filter (Discrete or Continuous)/1 -> Sum1/1, Scope2/1

== system MicrogridControl/BESS/BESS Integrated/Detailed/BESS Controller/Grid Forming/Power Control/ActivePowerControl/vsmControl ==
  note: Damping power input
  note: Measured power
  Pref : Inport
  Pmeas : Inport  Port=2
  fref : Inport  Port=3
  cntrlflag : Inport  Port=4
  fgrid : Inport  Port=5
  Add : Sum  Inputs=+-
  Constant2 : Constant  Value=pi/2
  Damping Frequency : Subsystem  Variant=on  VariantControlMode=label  VariantControl=Choice  LabelModeActiveChoice=constFreq
  Discrete-Time Integrator : DiscreteIntegrator  IntegratorMethod=Integration: Backward Euler  InitialCondition=1  SampleTime=activePowerSampleTime  LimitOutput=on  UpperSaturationLimit=1.1  LowerSaturationLimit=0.9  ICPrevOutput=DiscIntNeverNeededParam  ICPrevScaledInput=DiscIntNeverNeededParam
  Gain : Gain  Gain=powerFreq*2*pi
  Gain1 : Gain  Gain=1/vsmInertiaTC
  Gain2 : Gain  Gain=vsmDampingConst*powerFreq
  Integrator with Wrapped State (Discrete or Continuous) : eeGeneralControl/Integrator with Wrapped State (Discrete or Continuous)  LabelModeActiveChoice=Discrete  WrappedStateUpperValue=2*pi  WrappedStateLowerValue=0  x0=0  Ts=activePowerSampleTime
  Low-Pass Filter (Discrete or Continuous) : eeGeneralControl/Low-Pass Filter (Discrete or Continuous)  K=1  T=vsmPmeasFilterTC  B=inf  A=-inf  init_option=Specify as parameter  x0=0  Ts=activePowerSampleTime
  Power Reference Selection : Subsystem
  Saturation : Saturate  UpperLimit=dampingPowerMaxLimit  LowerLimit=dampingPowerMinLimit
  Scope : Scope
      settings: ActiveDisplayYMinimum=-1  ActiveDisplayYMaximum=1
  Sum1 : Sum  Inputs=-+-|
  Sum2 : Sum  Inputs=|+-
  Unit Delay : UnitDelay  SampleTime=-1  HasFrameUpgradeWarning=on
  Unit Delay1 : UnitDelay  SampleTime=-1  HasFrameUpgradeWarning=on
  Theta : Outport
  w : Outport  Port=2
  wires:
  [Wsm] -> Power Reference Selection/4(Wsm)
  Pmeas/1 -> Low-Pass Filter (Discrete or Continuous)/1
  fref/1 -> Power Reference Selection/3(fref)
  Pref/1 -> Power Reference Selection/2(Pref)
  cntrlflag/1 -> Power Reference Selection/1(cntrlflag)
  Damping Frequency/1(fmeas) -> Sum2/2
  fgrid/1 -> Damping Frequency/1(fref)
  Saturation/1 -> Sum1/3  "Pdamping"
  Unit Delay1/1 -> [Wsm]
  Unit Delay/1 -> Gain2/1
  Gain/1 -> w/1, Scope/1, Integrator with Wrapped State (Discrete or Continuous)/1
  Gain1/1 -> Discrete-Time Integrator/1
  Sum2/1 -> Unit Delay/1
  Power Reference Selection/1(power) -> Sum1/2
  Gain2/1 -> Saturation/1
  Low-Pass Filter (Discrete or Continuous)/1 -> Sum1/1
  Discrete-Time Integrator/1 -> Sum2/1, Unit Delay1/1, Gain/1
  Add/1 -> Theta/1
  Constant2/1 -> Add/2
  Sum1/1 -> Gain1/1  "Pinertia"
  Integrator with Wrapped State (Discrete or Continuous)/1 -> Add/1
